simulink model "CPI_P1_Primeira_Ordem_Simulink"  (R2024a)
settings: Solver=VariableStepAuto  StartTime=0.0  StopTime=10.0  RelTol=1e-3
undefined symbols (not defined in the file): den, den_a, den_MF, den_s, num, num_a, num_MF, num_s
settings Model: Creator=Carlos Augusto  LastModifiedBy=Carlos Augusto

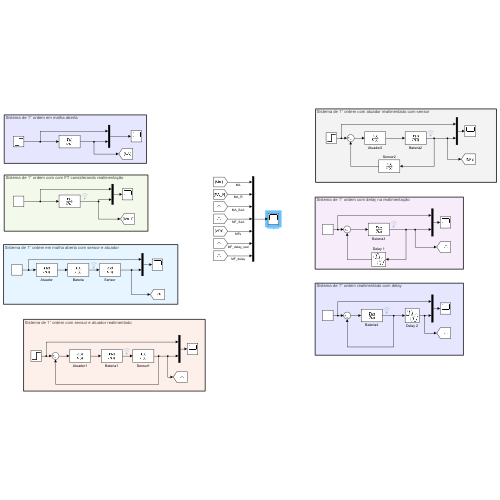
[thumbnail: Simulink's stored preview of the top-level diagram]
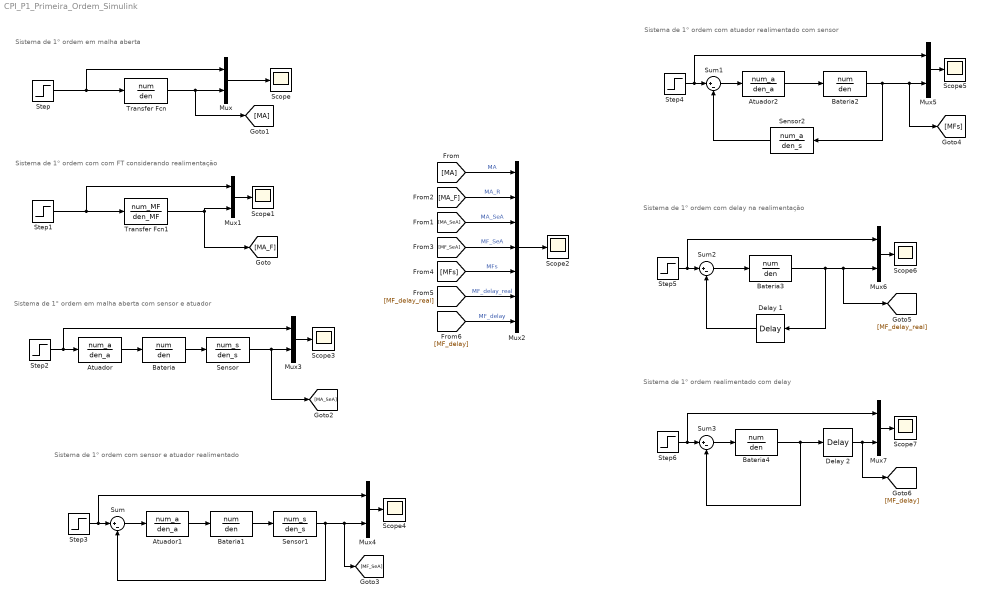
== system CPI_P1_Primeira_Ordem_Simulink ==
  note: Sistema de 1° ordem com delay na realimentação
  note: Sistema de 1° ordem com atuador realimentado com sensor
  note: Sistema de 1° ordem com sensor e atuador realimentado
  note: Sistema de 1° ordem em malha aberta com sensor e atuador
  note: Sistema de 1° ordem com com FT considerando realimentação
  note: Sistema de 1° ordem em malha aberta
  note: Sistema de 1° ordem realimentado com delay
  Atuador : TransferFcn  Numerator=num_a  Denominator=den_a
  Atuador1 : TransferFcn  Numerator=num_a  Denominator=den_a
  Atuador2 : TransferFcn  Numerator=num_a  Denominator=den_a
  Bateria{,1..4} (5 alike) : TransferFcn  Numerator=num  Denominator=den
  Delay 1 : TransportDelay  DelayTime=0.3
  Delay 2 : TransportDelay
  Mux{,1,3..7} (7 alike) : Mux  Inputs=2
  Mux2 : Mux  Inputs=7
  Scope{,1..7} (8 alike) : Scope
  Sensor : TransferFcn  Numerator=num_s  Denominator=den_s
  Sensor1 : TransferFcn  Numerator=num_s  Denominator=den_s
  Sensor2 : TransferFcn  Numerator=num_a  Denominator=den_s
  Step{,1..6} (7 alike) : Step  SampleTime=0
  Sum{,1..3} (4 alike) : Sum  Inputs=|+-
  Transfer Fcn : TransferFcn  Numerator=num  Denominator=den
  Transfer Fcn1 : TransferFcn  Numerator=num_MF  Denominator=den_MF
  wires:
  Step/1 -> Mux/1, Transfer Fcn/1
  Transfer Fcn/1 -> [MA], Mux/2
  Mux/1 -> Scope/1
  Transfer Fcn1/1 -> Mux1/2, [MA_F]
  Step1/1 -> Mux1/1, Transfer Fcn1/1
  Mux2/1 -> Scope2/1
  Step2/1 -> Mux3/1, Atuador/1
  Atuador/1 -> Bateria/1
  Bateria/1 -> Sensor/1
  Sensor/1 -> Mux3/2, [MA_SeA]
  Sensor1/1 -> Sum/2, Mux4/2, [MF_SeA]
  Atuador1/1 -> Bateria1/1
  Bateria1/1 -> Sensor1/1
  Sum/1 -> Atuador1/1
  Step3/1 -> Mux4/1, Sum/1
  [MA] -> Mux2/1  "MA"
  [MA_F] -> Mux2/2  "MA_R"
  [MA_SeA] -> Mux2/3  "MA_SeA"
  [MF_SeA] -> Mux2/4  "MF_SeA"
  Mux1/1 -> Scope1/1
  Mux3/1 -> Scope3/1
  Mux4/1 -> Scope4/1
  Sum1/1 -> Atuador2/1
  Step4/1 -> Mux5/1, Sum1/1
  Atuador2/1 -> Bateria2/1
  Mux5/1 -> Scope5/1
  Bateria2/1 -> Sensor2/1, [MFs], Mux5/2
  Sensor2/1 -> Sum1/2
  [MFs] -> Mux2/5  "MFs"
  Step5/1 -> Mux6/1, Sum2/1
  Sum2/1 -> Bateria3/1
  Mux6/1 -> Scope6/1
  Bateria3/1 -> Delay 1/1, Mux6/2, [MF_delay_real]
  Delay 1/1 -> Sum2/2
  [MF_delay_real] -> Mux2/6  "MF_delay_real"
  Sum3/1 -> Bateria4/1
  Bateria4/1 -> Delay 2/1, Sum3/2
  Mux7/1 -> Scope7/1
  Step6/1 -> Mux7/1, Sum3/1
  Delay 2/1 -> [MF_delay], Mux7/2
  [MF_delay] -> Mux2/7  "MF_delay"
